simulink model "OBALKA"  (R2023a)
settings: Solver=VariableStepAuto  StartTime=0.0  StopTime=15  RelTol=1e-3
settings Model: Creator=kaulejan  LastModifiedBy=MarekUser
settings SolverCC: AlgebraicLoopSolver=TrustRegion
settings DebuggingCC: UnconnectedInputMsg=warning  UnconnectedOutputMsg=warning  UnconnectedLineMsg=warning
settings ModelReferenceCC: EnableRefExpFcnMdlSchedulingChecks=on

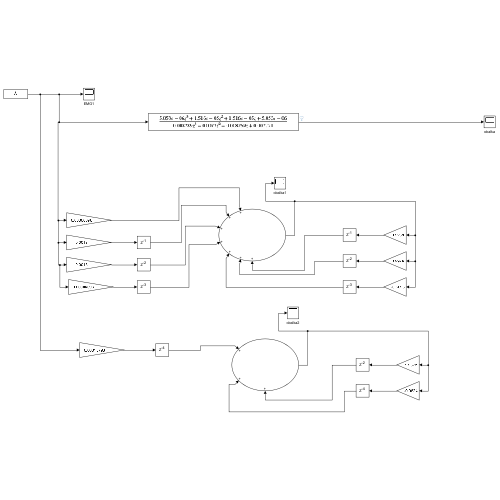
[thumbnail: Simulink's stored preview of the top-level diagram]
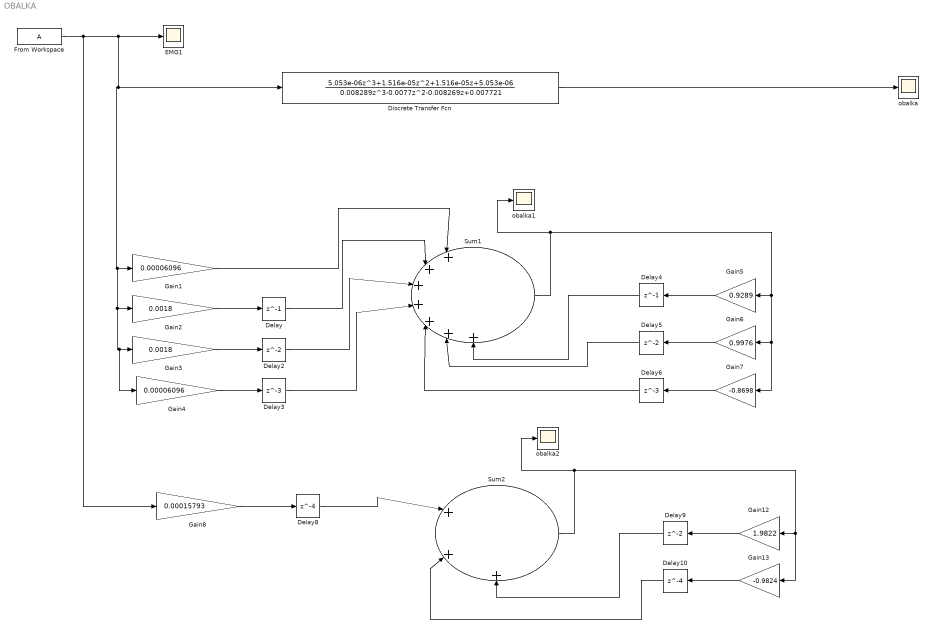
== system OBALKA ==
  Delay : Delay  DelayLength=1  SampleTime=0.002
  Delay10 : Delay  DelayLength=4  SampleTime=0.002
  Delay2 : Delay  SampleTime=0.002
  Delay3 : Delay  DelayLength=3  SampleTime=0.002
  Delay4 : Delay  DelayLength=1  SampleTime=0.002
  Delay5 : Delay  SampleTime=0.002
  Delay6 : Delay  DelayLength=3  SampleTime=0.002
  Delay8 : Delay  DelayLength=4  SampleTime=0.002
  Delay9 : Delay  SampleTime=0.002
  Discrete Transfer Fcn : DiscreteTransferFcn  Numerator=[5.053e-06 1.516e-05 1.516e-05 5.053e-06]  Denominator=[0.008289 -0.0077 -0.008269 0.007721]  SampleTime=0.002
  EMG1 : Scope
  From Workspace : FromWorkspace  VariableName=A  SampleTime=0.002
  Gain1 : Gain  Gain=0.00006096
  Gain12 : Gain  Gain=1.9822
  Gain13 : Gain  Gain=-0.9824
  Gain2 : Gain  Gain=0.0018
  Gain3 : Gain  Gain=0.0018
  Gain4 : Gain  Gain=0.00006096
  Gain5 : Gain  Gain=0.9289
  Gain6 : Gain  Gain=0.9976
  Gain7 : Gain  Gain=-0.8698
  Gain8 : Gain  Gain=0.00015793
  Sum1 : Sum  Inputs=|+++++++
  Sum2 : Sum  Inputs=|+++
  obalka : Scope
  obalka1 : Scope
  obalka2 : Scope
  wires:
  Discrete Transfer Fcn/1 -> obalka/1
  Gain1/1 -> Sum1/1
  Delay/1 -> Sum1/2
  Gain2/1 -> Delay/1
  Gain3/1 -> Delay2/1
  Delay2/1 -> Sum1/3
  Delay3/1 -> Sum1/4
  Gain4/1 -> Delay3/1
  Gain5/1 -> Delay4/1
  Gain6/1 -> Delay5/1
  Delay4/1 -> Sum1/7
  Delay5/1 -> Sum1/6
  Gain7/1 -> Delay6/1
  Delay6/1 -> Sum1/5
  Sum1/1 -> obalka1/1, Gain7/1, Gain6/1, Gain5/1
  From Workspace/1 -> Gain8/1, Discrete Transfer Fcn/1, Gain4/1, Gain3/1, Gain2/1, Gain1/1, EMG1/1
  Sum2/1 -> obalka2/1, Gain13/1, Gain12/1
  Gain13/1 -> Delay10/1
  Gain12/1 -> Delay9/1
  Gain8/1 -> Delay8/1
  Delay8/1 -> Sum2/1
  Delay9/1 -> Sum2/3
  Delay10/1 -> Sum2/2
